simulink model "sample01_current"  (R2023a)
settings: Solver=ode1  StartTime=0.0  StopTime=inf  FixedStep=0.005  RelTol=1e-3  EnableMultiTasking=on
libraries: arduinolib x4, simulink x1
settings Model: ExtModeTrigDuration=2  Creator=kawata  LastModifiedBy=kawata
settings SolverCC: AutoInsertRateTranBlk=on
settings DataIOCC: ReturnWorkspaceOutputs=off
settings OptimizationCC: EnhancedBackFolding=on  PassReuseOutputArgsAs=Individual arguments  ZeroExternalMemoryAtStartup=off  ZeroInternalMemoryAtStartup=off  MaxStackSize=64  OptimizeBlockOrder=speed  DifferentSizesBufferReuse=on  OptimizationCustomize=off  EfficientTunableParamExpr=on
settings DebuggingCC: ParameterTunabilityLossMsg=error
settings HardwareCC: ProdBitPerInt=16  ProdBitPerPointer=16  ProdBitPerSizeT=16  ProdBitPerPtrDiffT=16  ProdLargestAtomicFloat=None  ProdWordSize=8  ProdHWDeviceType=Atmel->AVR  UseEmbeddedCoderFeatures=off  UseSimulinkCoderFeatures=off
settings SFSimCC: MATLABDynamicMemAlloc=off
settings RTWCC: Description=Embedded Coder  SystemTargetFile=ert.tlc  HardwareBoard=Arduino Uno  TemplateMakefile=ert_default_tmf  Toolchain=Arduino AVR  BuildConfiguration=Faster Runs  GPUComputeCapability=5.0
settings CodeAppCC: ForceParamTrailComments=on  IgnoreCustomStorageClasses=off  OperatorAnnotations=on  SimulinkDataObjDesc=on  SFDataObjDesc=on  InsertBlockDesc=on
settings ERTTargetCC: SupportContinuousTime=on  SupportNonInlinedSFcns=on  SupportVariableSizeSignals=on  ExtModeTransport=3  ExtModeStaticAlloc=on  ExtModeAutomaticAllocSize=off  ExtModeStaticAllocSize=250  ExtModeMexFile=ext_xcp  ExtModeIntrfLevel=Level2 - Open

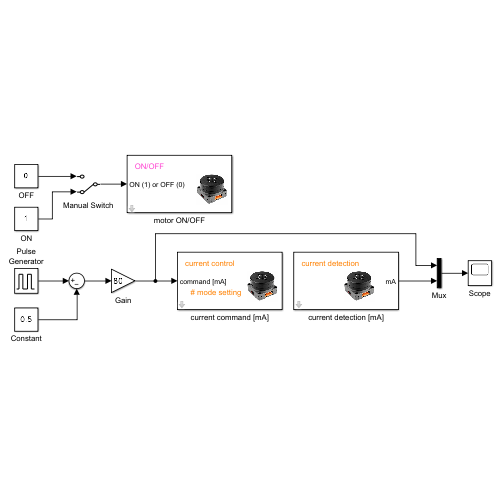
[thumbnail: Simulink's stored preview of the top-level diagram]
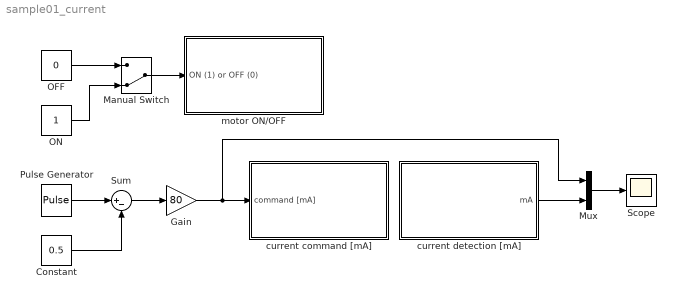
== system sample01_current ==
  Constant : Constant  Value=0.5
  Gain : Gain  Gain=80
  Manual Switch : ManualSwitch  CurrentSetting=0
  Mux : Mux  Inputs=2
  OFF : Constant  Value=0
  ON : Constant
  Pulse Generator : DiscretePulseGenerator  PulseType=Time based  Period=4  PulseWidth=50  PhaseDelay=1
  Scope : Scope
  Sum : Sum  Inputs=|+-
  current command [mA] : Subsystem  mask(current command [A]){I2CAddress=0x64}
      mask prompts: I2CAddress "I2C Address"
      mask help:
      | current mode
      | ---------------------------------
      | PID gain of current controller
      |  P: 0.002
      |  I: 0.00005
      |  D: 0
      | ---------------------------------
      | Changing the PID gains is not permitted.
      mask DialogControl ParameterGroupVar Prompt: パラメーター
      mask Display:
      | image('roller485.png', [55,10,75,56]);
      | color('orange');
      | text(10, 60, 'current control');
      | text(17, 22, '# mode setting');
  current detection [mA] : Subsystem  mask{I2CAddress=0x64, sample_time=0.005}
      mask prompts: I2CAddress "I2C Address"; sample_time "Sample Time"
      mask DialogControl ParameterGroupVar Prompt: パラメーター
      mask Display:
      | image('roller485.png', [30,10,75,56]);
      | color('orange');
      | text(10, 60, 'current detection');
  motor ON/OFF : Subsystem  mask{I2CAddress=0x64}
      mask prompts: I2CAddress "I2C Address"
      mask help:
      | 0: motor off
      | 1: motor on
      mask DialogControl ParameterGroupVar Prompt: パラメーター
      mask Display:
      | image('roller485.png', [55,10,75,56]);
      | color('magenta');
      | text(10, 60, 'ON/OFF');
  wires:
  Manual Switch/1 -> motor ON/OFF/1(ON (1) or OFF (0))
  OFF/1 -> Manual Switch/1
  ON/1 -> Manual Switch/2
  Gain/1 -> current command [mA]/1(command [mA]), Mux/1
  Sum/1 -> Gain/1
  Constant/1 -> Sum/2
  Pulse Generator/1 -> Sum/1
  current detection [mA]/1(mA) -> Mux/2
  Mux/1 -> Scope/1

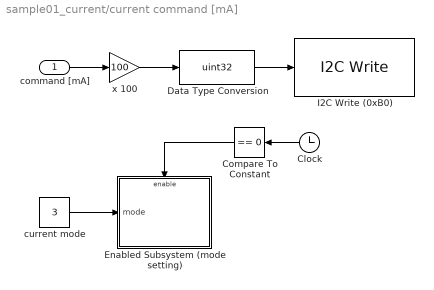
== system sample01_current/current command [mA] ==
  command [mA] : Inport
  "Clock " : Clock
  Compare To Constant : simulink/Logic and Bit Operations/Compare To Constant  relop===  const=0  OutDataTypeStr=boolean
  Data Type Conversion : DataTypeConversion  OutDataTypeStr=uint32  SaturateOnIntegerOverflow=off  RndMeth=Floor
  Enabled Subsystem (mode setting) : Subsystem  TreatAsAtomicUnit=on
  I2C Write (0xB0) : arduinolib/I2C Write  I2CModule=0  Mode=Master  SlaveAddress=I2CAddress  SlaveByteOrder=LittleEndian  Direction=Transmitter  RegisterAddressMode=on  RegisterAddress=0xB0  SlaveDataType=uint8  DataLength=1  NoAck=off  RepeatedStart=off  OutputStatus=off  blockPlatform=ARDUINO
  current mode : Constant  Value=3
  x 100 : Gain  Gain=100
  wires:
  x 100/1 -> Data Type Conversion/1
  command [mA]/1 -> x 100/1
  Data Type Conversion/1 -> I2C Write (0xB0)/1
  "Clock "/1 -> Compare To Constant/1
  Compare To Constant/1 -> Enabled Subsystem (mode setting)/Enable
  current mode/1 -> Enabled Subsystem (mode setting)/1(mode)

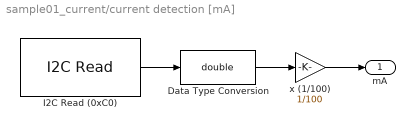
== system sample01_current/current detection [mA] ==
  Data Type Conversion : DataTypeConversion  OutDataTypeStr=double  SaturateOnIntegerOverflow=off  RndMeth=Floor
  I2C Read (0xC0) : arduinolib/I2C Read  I2CModule=0  Mode=Master  SlaveAddress=0x64  SlaveByteOrder=LittleEndian  Direction=Receiver  RegisterAddressMode=on  RegisterAddress=0xC0  SlaveDataType=int32  DataLength=1  NoAck=off  RepeatedStart=off  OutputStatus=off  blockPlatform=ARDUINO  SampleTime=sample_time
  x (1/100) : Gain  Gain=1/100
  mA : Outport
  wires:
  Data Type Conversion/1 -> x (1/100)/1
  x (1/100)/1 -> mA/1
  I2C Read (0xC0)/1 -> Data Type Conversion/1

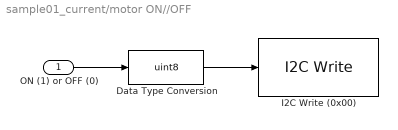
== system sample01_current/motor ON//OFF ==
  ON (1) or OFF (0) : Inport
  Data Type Conversion : DataTypeConversion  OutDataTypeStr=uint8  SaturateOnIntegerOverflow=off  RndMeth=Floor
  I2C Write (0x00) : arduinolib/I2C Write  I2CModule=0  Mode=Master  SlaveAddress=I2CAddress  SlaveByteOrder=BigEndian  Direction=Transmitter  RegisterAddressMode=on  RegisterAddress=0x00  SlaveDataType=uint8  DataLength=1  NoAck=off  RepeatedStart=off  OutputStatus=off  blockPlatform=ARDUINO
  wires:
  Data Type Conversion/1 -> I2C Write (0x00)/1
  ON (1) or OFF (0)/1 -> Data Type Conversion/1

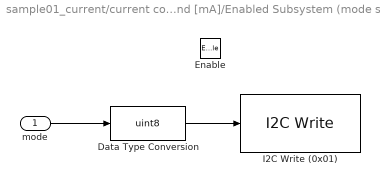
== system sample01_current/current command [mA]/Enabled Subsystem (mode setting) ==
  mode : Inport
  Enable : EnablePort
  Data Type Conversion : DataTypeConversion  OutDataTypeStr=uint8  SaturateOnIntegerOverflow=off  RndMeth=Floor
  I2C Write (0x01) : arduinolib/I2C Write  I2CModule=0  Mode=Master  SlaveAddress=I2CAddress  SlaveByteOrder=BigEndian  Direction=Transmitter  RegisterAddressMode=on  RegisterAddress=0x01  SlaveDataType=uint8  DataLength=1  NoAck=off  RepeatedStart=off  OutputStatus=off  blockPlatform=ARDUINO
  wires:
  Data Type Conversion/1 -> I2C Write (0x01)/1
  mode/1 -> Data Type Conversion/1
